simulink model "test_snap_dram_circ"  (Simulink 7.2)
settings: Solver=ode45  StartTime=0.0  StopTime=12000  RelTol=1e-3
libraries: xbsIndex_r4 x91, xps_library x7, casper_library_misc x5
settings Model: Creator=dsp  LastModifiedBy=root
settings OptimizationCC: InitFltsAndDblsToZero=on
settings DebuggingCC: SaveWithParameterizedLinksMsg=none  SignalResolutionControl=TryResolveAllWithWarning  MultiTaskDSMMsg=warning  MultiTaskCondExecSysMsg=none  StrictBusMsg=None
settings RTWCC: IncludeERTFirstTime=on
settings GRTTargetCC: TargetFcnLib=ansi_tfl_tmw.mat

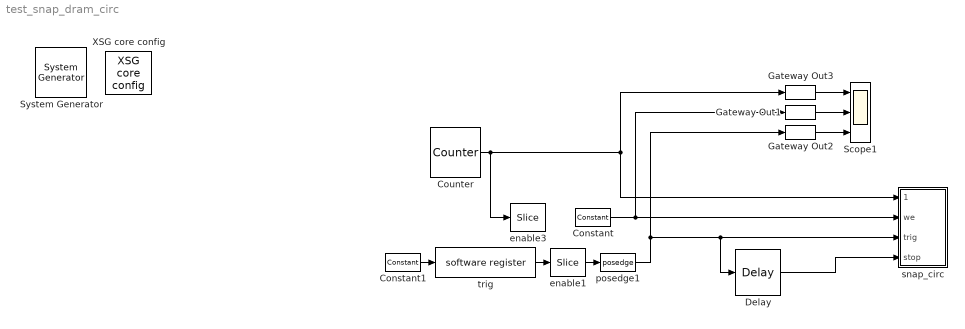
== system test_snap_dram_circ ==
  " System Generator" : xbsIndex_r4/ System Generator  Tag=genX  SystemSampleTime=-1  xilinxfamily=virtex5  part=xc5vsx95t  speed=-1  package=ff1136  synthesis_tool=XST  clock_wrapper=Clock Enables  directory=./test_snap_dram_circ/sysgen  testbench=off  simulink_period=1  sysclk_period=10  dcm_input_clock_period=100  incr_netlist=off  trim_vbits=Everywhere in SubSystem  dbl_ovrd=According to Block Masks  core_generation=According to Block Masks  run_coregen=off  deprecated_control=off  eval_field=0  block_type=sysgen
      settings: block_version=10.1.3
  Constant : xbsIndex_r4/Constant  arith_type=Boolean  const=1  n_bits=1  bin_pt=0  explicit_period=on  period=1  equ=P=C  opselect=C  inp2=PCIN>>17  opr=+  inp1=P  carry=CIN  dbl_ovrd=off  block_type=constant
  Constant1 : xbsIndex_r4/Constant  arith_type=Boolean  const=1  n_bits=1  bin_pt=0  explicit_period=on  period=1  equ=P=C  opselect=C  inp2=PCIN>>17  opr=+  inp1=P  carry=CIN  dbl_ovrd=off  block_type=constant
  Counter : xbsIndex_r4/Counter  cnt_type=Free Running  cnt_to=Inf  operation=Up  start_count=0  cnt_by_val=1  arith_type=Unsigned  n_bits=64  bin_pt=0  load_pin=off  rst=off  en=off  explicit_period=on  period=1  dbl_ovrd=off  use_behavioral_HDL=off  implementation=Fabric  use_rpm=on  block_type=counter
      settings: xl_area=[0, 0, 0, 0, 0, 0, 0]
  Delay : xbsIndex_r4/Delay  en=off  latency=5200  dbl_ovrd=off  reg_retiming=off  block_type=delay
      settings: xl_area=[0, 0, 0, 0, 0, 0, 0]
  Gateway Out1 : xbsIndex_r4/Gateway Out  hdl_port=off  timing_constraint=None  locs_specified=off  LOCs={}  block_type=gatewayout
      settings: infoedit="Gateway out block.  Converts Xilinx fixed point inputs into ouputs of type Simulink integer, double, or fixed point.<P><P>Hardware notes:  In hardware these blocks become top level output ports or are discarded, depending on how they are configured."  xl_area=[0, 0, 0, 0, 0, 0, 0]  block_version=10.1.3
  Gateway Out2 : xbsIndex_r4/Gateway Out  hdl_port=off  timing_constraint=None  locs_specified=off  LOCs={}  block_type=gatewayout
      settings: infoedit="Gateway out block.  Converts Xilinx fixed point inputs into ouputs of type Simulink integer, double, or fixed point.<P><P>Hardware notes:  In hardware these blocks become top level output ports or are discarded, depending on how they are configured."  xl_area=[0, 0, 0, 0, 0, 0, 0]  block_version=10.1.3
  Gateway Out3 : xbsIndex_r4/Gateway Out  hdl_port=off  timing_constraint=None  locs_specified=off  LOCs={}  block_type=gatewayout
      settings: infoedit="Gateway out block.  Converts Xilinx fixed point inputs into ouputs of type Simulink integer, double, or fixed point.<P><P>Hardware notes:  In hardware these blocks become top level output ports or are discarded, depending on how they are configured."  xl_area=[0, 0, 0, 0, 0, 0, 0]  block_version=10.1.3
  Scope1 : Scope  NumInputPorts=3
      settings: YMin=272014000~0~0  YMax=300648000~110~1
  XSG core config : xps_library/XSG core config  Tag=xps:xsg  SystemSampleTime=-1  hw_sys=ROACH:sx95t  ibob_linux=off  clk_src=sys_clk  iBOB_clk_src=sys_clk  BEE2_ctrl_clk_src=sys_clk  BEE2_usr_clk_src=sys_clk  ROACH_clk_src=sys_clk  CORR_clk_src=sys_clk  gpio_clk_io_group=iBOB:sma  gpio_clk_bit_index=0  clk_rate=100  sample_period=1  synthesis_tool=XST  mpc_type=powerpc440_ext
  enable1 : xbsIndex_r4/Slice  nbits=1  boolean_output=on  mode=Lower Bit Location + Width  bit1=0  base1=LSB of Input  bit0=0  base0=LSB of Input  dbl_ovrd=off  block_type=slice
      settings: infoedit="Extracts a given range of bits from each input sample and presents it at the output.  The output type is ordinarily unsigned with binary point at zero, but can be Boolean when the slice is one bit wide.<P><P>Hardware notes: In hardware this block costs nothing."  block_version=10.1.3
  enable3 : xbsIndex_r4/Slice  nbits=1  boolean_output=on  mode=Lower Bit Location + Width  bit1=0  base1=LSB of Input  bit0=0  base0=LSB of Input  dbl_ovrd=off  block_type=slice
      settings: infoedit="Extracts a given range of bits from each input sample and presents it at the output.  The output type is ordinarily unsigned with binary point at zero, but can be Boolean when the slice is one bit wide.<P><P>Hardware notes: In hardware this block costs nothing."  block_version=10.1.3
  posedge1 : casper_library_misc/posedge  Tag=Rising Edge Detector  SystemSampleTime=-1
  snap_circ : Subsystem  mask(snap_circ){nsamples=29}
      mask prompts: nsamples "Number of Samples (2^?)"
      mask help:
      | Backwards compatible with the normal snap block, but with the following upgrades:
      |  1) Ability to offset the trigger. Optionally delay the fabric trigger by a user-specified number of valids.
      |  2) 'Addr' register's MSb now indicates 'busy capturing'.
      |  3) Ability to capture continuously until a stop pulse is received. Data is captured into BRAM continuously, with old data being overwritten until a stop command is received. Then stop capturing when memory is filled. This enables you to get some data before and some data after the stop pulse. Use the 'tr_en_cnt' register to determine where you are in your vector.
  trig : xps_library/software register  Tag=xps:sw_reg  SystemSampleTime=-1  io_dir=From Processor  arith_type=Unsigned  bitwidth=32  bin_pt=0  sample_period=1  gw_name=test_snap_dram_circ_trig_user_data_out
      link override test_snap_circ_trig_user_data_out: arith_type=Unsigned  n_bits=32  bin_pt=0  period=1
  wires:
  Counter/1 -> Gateway Out3/1, snap_circ/1(data_in), enable3/1
  trig/1 -> enable1/1
  posedge1/1 -> Gateway Out2/1, Delay/1, snap_circ/3(trig)
  Gateway Out2/1 -> Scope1/3
  Gateway Out1/1 -> Scope1/2
  Gateway Out3/1 -> Scope1/1
  Constant1/1 -> trig/1
  enable1/1 -> posedge1/1
  Delay/1 -> snap_circ/4(stop)
  Constant/1 -> Gateway Out1/1, snap_circ/2(we)

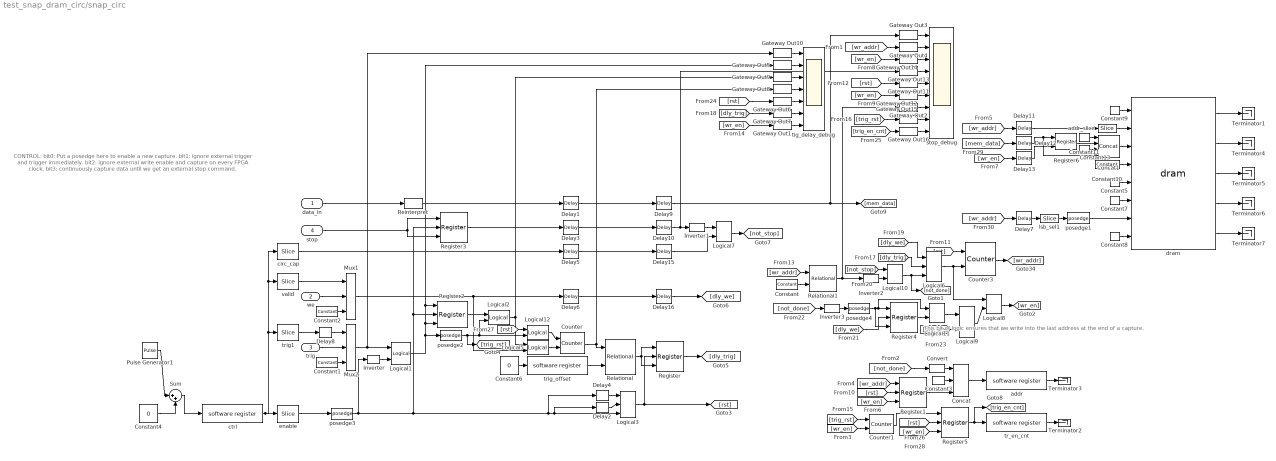
== system test_snap_dram_circ/snap_circ ==
  note: CONTROL:
      | bit0: Put a posedge here to enable a new capture.
      | bit1: ignore external trigger and trigger immediately.
      | bit2: ignore external write enable and capture on every FPGA clock.
      | bit3: continuously capture data until we get an external stop command.
  note: This bit of logic ensures that we
      | write into the last address
      | at the end of a capture.
  data_in : Inport  OutDataType=sfix(16)  OutScaling=2^0
  we : Inport  Port=2  OutDataType=sfix(16)  OutScaling=2^0
  trig : Inport  Port=3  OutDataType=sfix(16)  OutScaling=2^0
  stop : Inport  Port=4  OutDataType=sfix(16)  OutScaling=2^0
  Concat : xbsIndex_r4/Concat  num_inputs=3  dbl_ovrd=off  block_type=concat
      settings: block_version=10.1.3
  Concat1 : xbsIndex_r4/Concat  num_inputs=4  dbl_ovrd=off  block_type=concat
      settings: block_version=10.1.3
  Constant : xbsIndex_r4/Constant  arith_type=Unsigned  const=(2^nsamples)-1  n_bits=nsamples  bin_pt=0  explicit_period=on  period=1  equ=P=C  opselect=C  inp2=PCIN>>17  opr=+  inp1=P  carry=CIN  dbl_ovrd=off  block_type=constant
  Constant1 : xbsIndex_r4/Constant  arith_type=Boolean  const=1  n_bits=1  bin_pt=0  explicit_period=on  period=1  equ=P=C  opselect=C  inp2=PCIN>>17  opr=+  inp1=P  carry=CIN  dbl_ovrd=off  block_type=constant
  Constant10 : xbsIndex_r4/Constant  arith_type=Unsigned  const=2^32-1  n_bits=18  bin_pt=0  explicit_period=on  period=1  equ=P=C  opselect=C  inp2=PCIN>>17  opr=+  inp1=P  carry=CIN  dbl_ovrd=off  block_type=constant
  Constant11 : xbsIndex_r4/Constant  arith_type=Unsigned  const=0  n_bits=(144-128)/2  bin_pt=0  explicit_period=on  period=1  equ=P=C  opselect=C  inp2=PCIN>>17  opr=+  inp1=P  carry=CIN  dbl_ovrd=off  block_type=constant
  Constant13 : xbsIndex_r4/Constant  arith_type=Unsigned  const=0  n_bits=(144-128)/2  bin_pt=0  explicit_period=on  period=1  equ=P=C  opselect=C  inp2=PCIN>>17  opr=+  inp1=P  carry=CIN  dbl_ovrd=off  block_type=constant
  Constant2 : xbsIndex_r4/Constant  arith_type=Boolean  const=1  n_bits=1  bin_pt=0  explicit_period=on  period=1  equ=P=C  opselect=C  inp2=PCIN>>17  opr=+  inp1=P  carry=CIN  dbl_ovrd=off  block_type=constant
  Constant3 : xbsIndex_r4/Constant  arith_type=Unsigned  const=0  n_bits=32-nsamples-1  bin_pt=0  explicit_period=on  period=1  equ=P=C  opselect=C  inp2=PCIN>>17  opr=+  inp1=P  carry=CIN  dbl_ovrd=off  block_type=constant
  Constant4 : Constant  Value=0  OutDataType=sfix(16)  OutScaling=2^0
  Constant5 : xbsIndex_r4/Constant  arith_type=Boolean  const=0  n_bits=nsamples  bin_pt=0  explicit_period=on  period=1  equ=P=C  opselect=C  inp2=PCIN>>17  opr=+  inp1=P  carry=CIN  dbl_ovrd=off  block_type=constant
  Constant6 : Constant  Value=0  OutDataType=sfix(16)  OutScaling=2^0
  Constant7 : xbsIndex_r4/Constant  arith_type=Unsigned  const=0  n_bits=8  bin_pt=0  explicit_period=on  period=1  equ=P=C  opselect=C  inp2=PCIN>>17  opr=+  inp1=P  carry=CIN  dbl_ovrd=off  block_type=constant
  Constant8 : xbsIndex_r4/Constant  arith_type=Boolean  const=1  n_bits=nsamples  bin_pt=0  explicit_period=on  period=1  equ=P=C  opselect=C  inp2=PCIN>>17  opr=+  inp1=P  carry=CIN  dbl_ovrd=off  block_type=constant
  Constant9 : xbsIndex_r4/Constant  arith_type=Boolean  const=0  n_bits=nsamples  bin_pt=0  explicit_period=on  period=1  equ=P=C  opselect=C  inp2=PCIN>>17  opr=+  inp1=P  carry=CIN  dbl_ovrd=off  block_type=constant
  Convert : xbsIndex_r4/Convert  arith_type=Unsigned  n_bits=1  bin_pt=0  quantization=Truncate  overflow=Wrap  latency=0  dbl_ovrd=off  pipeline=off  block_type=convert
      settings: block_version=10.1.3
  Counter : xbsIndex_r4/Counter  cnt_type=Free Running  cnt_to=Inf  operation=Up  start_count=0  cnt_by_val=1  arith_type=Unsigned  n_bits=32  bin_pt=0  load_pin=off  rst=on  en=on  explicit_period=on  period=1  dbl_ovrd=off  use_behavioral_HDL=off  implementation=Fabric  use_rpm=on  block_type=counter
      settings: xl_area=[0, 0, 0, 0, 0, 0, 0]
  Counter1 : xbsIndex_r4/Counter  cnt_type=Free Running  cnt_to=Inf  operation=Up  start_count=0  cnt_by_val=1  arith_type=Unsigned  n_bits=32  bin_pt=0  load_pin=off  rst=on  en=on  explicit_period=on  period=1  dbl_ovrd=off  use_behavioral_HDL=off  implementation=Fabric  use_rpm=on  block_type=counter
      settings: xl_area=[0, 0, 0, 0, 0, 0, 0]
  Counter3 : xbsIndex_r4/Counter  cnt_type=Free Running  cnt_to=1  operation=Up  start_count=0  cnt_by_val=1  arith_type=Unsigned  n_bits=nsamples  bin_pt=0  load_pin=off  rst=on  en=on  explicit_period=on  period=1  dbl_ovrd=off  use_behavioral_HDL=off  implementation=Fabric  use_rpm=on  block_type=counter
      settings: xl_area=[0, 0, 0, 0, 0, 0, 0]
  Delay{1,3..7,9..13,15..16} (13 alike) : xbsIndex_r4/Delay  en=off  latency=1  dbl_ovrd=off  reg_retiming=on  block_type=delay
      settings: xl_area=[0, 0, 0, 0, 0, 0, 0]
  Delay2 : xbsIndex_r4/Delay  en=off  latency=2  dbl_ovrd=off  reg_retiming=on  block_type=delay
      settings: xl_area=[0, 0, 0, 0, 0, 0, 0]
  Delay8 : xbsIndex_r4/Delay  en=off  latency=3  dbl_ovrd=off  reg_retiming=on  block_type=delay
      settings: xl_area=[0, 0, 0, 0, 0, 0, 0]
  Gateway Out{1..16} (16 alike) : xbsIndex_r4/Gateway Out  hdl_port=off  timing_constraint=None  locs_specified=off  LOCs={}  block_type=gatewayout
      settings: infoedit="Gateway out block.  Converts Xilinx fixed point inputs into ouputs of type Simulink integer, double, or fixed point.<P><P>Hardware notes:  In hardware these blocks become top level output ports or are discarded, depending on how they are configured."  xl_area=[0, 0, 0, 0, 0, 0, 0]  block_version=10.1.3
  Inverter{,1..3} (4 alike) : xbsIndex_r4/Inverter  en=off  latency=0  dbl_ovrd=off  block_type=inv
      settings: xl_area=[0, 0, 0, 0, 0, 0, 0]
  Logical{1,5,7,9} (4 alike) : xbsIndex_r4/Logical  logical_function=AND  inputs=2  en=off  latency=0  precision=Full  arith_type=Unsigned  n_bits=8  bin_pt=2  align_bp=on  dbl_ovrd=off  block_type=logical
      settings: xl_area=[0, 0, 0, 0, 0, 0, 0]
  Logical{2,8,10..12} (5 alike) : xbsIndex_r4/Logical  logical_function=OR  inputs=2  en=off  latency=0  precision=Full  arith_type=Unsigned  n_bits=8  bin_pt=2  align_bp=on  dbl_ovrd=off  block_type=logical
      settings: xl_area=[0, 0, 0, 0, 0, 0, 0]
  Logical3 : xbsIndex_r4/Logical  logical_function=OR  inputs=3  en=off  latency=0  precision=Full  arith_type=Unsigned  n_bits=8  bin_pt=2  align_bp=on  dbl_ovrd=off  block_type=logical
      settings: xl_area=[0, 0, 0, 0, 0, 0, 0]
  Logical6 : xbsIndex_r4/Logical  logical_function=AND  inputs=3  en=off  latency=0  precision=Full  arith_type=Unsigned  n_bits=8  bin_pt=2  align_bp=on  dbl_ovrd=off  block_type=logical
      settings: xl_area=[0, 0, 0, 0, 0, 0, 0]
  Mux1 : xbsIndex_r4/Mux  inputs=2  en=off  latency=0  precision=Full  arith_type="Signed  (2's comp)"  n_bits=8  bin_pt=2  quantization=Truncate  overflow=Wrap  dbl_ovrd=off  block_type=mux
      settings: xl_area=[0, 0, 0, 0, 0, 0, 0]
  Mux2 : xbsIndex_r4/Mux  inputs=2  en=off  latency=0  precision=Full  arith_type="Signed  (2's comp)"  n_bits=8  bin_pt=2  quantization=Truncate  overflow=Wrap  dbl_ovrd=off  block_type=mux
      settings: xl_area=[0, 0, 0, 0, 0, 0, 0]
  Pulse Generator1 : DiscretePulseGenerator  Period=4096  PulseWidth=2
  Register{,1..5} (6 alike) : xbsIndex_r4/Register  init=0  rst=on  en=on  dbl_ovrd=off  block_type=register
      settings: xl_area=[0, 0, 0, 0, 0, 0, 0]
  Register6 : xbsIndex_r4/Register  init=0  rst=off  en=on  dbl_ovrd=off  block_type=register
  Reinterpret : xbsIndex_r4/Reinterpret  force_arith_type=on  arith_type=Unsigned  force_bin_pt=on  bin_pt=0  block_type=reinterpret
      settings: infoedit="Changes signal type without altering the binary representation.   You can changed the signal between signed and unsigned, and relocate the binary point.<P><P>Hardware notes: In hardware this block costs nothing.<P><P>Example:  Suppose the input is 6 bits wide, signed, with 2 fractional bits, and the output is forced to unsigned with 0 fractional bits.  Then an input of -2.0 (1110.00 in binary 2's complement) becomes an output of 56 (111000 in binary)."  block_version=10.1.3
  Relational : xbsIndex_r4/Relational  mode=a>b  en=off  latency=0  dbl_ovrd=off  block_type=relational
      settings: xl_area=[0, 0, 0, 0, 0, 0, 0]  block_version=10.1.3
  Relational1 : xbsIndex_r4/Relational  mode=a>=b  en=off  latency=0  dbl_ovrd=off  block_type=relational
      settings: xl_area=[0, 0, 0, 0, 0, 0, 0]  block_version=10.1.3
  Sum : Sum  Inputs=|++  OutDataType=sfix(16)  OutScaling=2^0
  Terminator{1..7} (7 alike) : Terminator
  addr : xps_library/software register  Tag=xps:sw_reg  SystemSampleTime=-1  io_dir=To Processor  arith_type=Unsigned  bitwidth=32  bin_pt=0  sample_period=1  gw_name=test_snap_dram_circ_snap_circ_addr_user_data_in
      link override convert: arith_type=Unsigned  n_bits=32  bin_pt=0
  addr_slice : xbsIndex_r4/Slice  nbits=72  boolean_output=off  mode=Two Bit Locations  bit1=0  base1=MSB of Input  bit0=2  base0=LSB of Input  dbl_ovrd=off  block_type=slice
      settings: block_version=10.1.3
  circ_cap : xbsIndex_r4/Slice  nbits=1  boolean_output=on  mode=Lower Bit Location + Width  bit1=0  base1=LSB of Input  bit0=3  base0=LSB of Input  dbl_ovrd=off  block_type=slice
      settings: infoedit="Extracts a given range of bits from each input sample and presents it at the output.  The output type is ordinarily unsigned with binary point at zero, but can be Boolean when the slice is one bit wide.<P><P>Hardware notes: In hardware this block costs nothing."  block_version=10.1.3
  ctrl : xps_library/software register  Tag=xps:sw_reg  SystemSampleTime=-1  io_dir=From Processor  arith_type=Unsigned  bitwidth=32  bin_pt=0  sample_period=1  gw_name=test_snap_dram_circ_snap_circ_ctrl_user_data_out
      link override r_4f_2x_16a_r322d_snap_descramble0_ctrl_user_data_out: arith_type=Unsigned  n_bits=32  bin_pt=0  period=1
      link override test_snap2_10_1_snap_circ_ctrl_user_data_out: arith_type=Unsigned  n_bits=32  bin_pt=0  period=1
      link override test_snap_circ_snap_circ_ctrl_user_data_out: arith_type=Unsigned  n_bits=32  bin_pt=0  period=1
  dram : xps_library/dram  Tag=xps:dram  SystemSampleTime=-1  dimm=1  arith_type=Unsigned  bin_pt=0  ip_clock=200  sample_period=1  bram_fifos=on  disable_tag=on  use_sim=off  ram_depth=18  bank_mgt=off  wide_data=off  half_burst=off  use_sniffer=on
      link override convert_data_in: arith_type=Unsigned  n_bits=144  bin_pt=0
      link override convert_wr_be: n_bits=18
      link override force_rd_dout: arith_type=Unsigned  bin_pt=0
      link override sim_wrapper/dram_sim: sim_method=Inactive  engine_block=ModelSim
      link override test_snap_dram_snap_circ_dram_Mem_Rd_Dout: n_bits=144
  enable : xbsIndex_r4/Slice  nbits=1  boolean_output=on  mode=Lower Bit Location + Width  bit1=0  base1=LSB of Input  bit0=0  base0=LSB of Input  dbl_ovrd=off  block_type=slice
      settings: infoedit="Extracts a given range of bits from each input sample and presents it at the output.  The output type is ordinarily unsigned with binary point at zero, but can be Boolean when the slice is one bit wide.<P><P>Hardware notes: In hardware this block costs nothing."  block_version=10.1.3
  lsb_sel1 : xbsIndex_r4/Slice  nbits=1  boolean_output=on  mode=Lower Bit Location + Width  bit1=0  base1=LSB of Input  bit0=0  base0=LSB of Input  dbl_ovrd=off  block_type=slice
      settings: infoedit="Extracts a given range of bits from each input sample and presents it at the output.  The output type is ordinarily unsigned with binary point at zero, but can be Boolean when the slice is one bit wide.<P><P>Hardware notes: In hardware this block costs nothing."  block_version=10.1.3
  posedge{1..4} (4 alike) : casper_library_misc/posedge  Tag=Rising Edge Detector  SystemSampleTime=-1
  stop_debug : Scope  NumInputPorts=9
      settings: YMin=2.72014e+008~0~0~-5~-5~-5~-5~-5~-5  YMax=3.00648e+008~110~1~5~5~5~5~5~5  SaveName=ScopeData12
  tig_delay_debug : Scope  NumInputPorts=7
      settings: YMin=2.72014e+008~0~0~-5~-5~-5~-5  YMax=3.00648e+008~110~1~5~5~5~5  SaveName=ScopeData16
  tr_en_cnt : xps_library/software register  Tag=xps:sw_reg  SystemSampleTime=-1  io_dir=To Processor  arith_type=Unsigned  bitwidth=32  bin_pt=0  sample_period=1  gw_name=test_snap_dram_circ_snap_circ_tr_en_cnt_user_data_in
      link override convert: arith_type=Unsigned  n_bits=32  bin_pt=0
  trig1 : xbsIndex_r4/Slice  nbits=1  boolean_output=on  mode=Lower Bit Location + Width  bit1=0  base1=LSB of Input  bit0=1  base0=LSB of Input  dbl_ovrd=off  block_type=slice
      settings: infoedit="Extracts a given range of bits from each input sample and presents it at the output.  The output type is ordinarily unsigned with binary point at zero, but can be Boolean when the slice is one bit wide.<P><P>Hardware notes: In hardware this block costs nothing."  block_version=10.1.3
  trig_offset : xps_library/software register  Tag=xps:sw_reg  SystemSampleTime=-1  io_dir=From Processor  arith_type=Unsigned  bitwidth=32  bin_pt=0  sample_period=1  gw_name=test_snap_dram_circ_snap_circ_trig_offset_user_data_out
      link override test_snap_circ_snap_circ_trig_offset_user_data_out: arith_type=Unsigned  n_bits=32  bin_pt=0  period=1
  valid : xbsIndex_r4/Slice  nbits=1  boolean_output=on  mode=Lower Bit Location + Width  bit1=0  base1=LSB of Input  bit0=2  base0=LSB of Input  dbl_ovrd=off  block_type=slice
      settings: infoedit="Extracts a given range of bits from each input sample and presents it at the output.  The output type is ordinarily unsigned with binary point at zero, but can be Boolean when the slice is one bit wide.<P><P>Hardware notes: In hardware this block costs nothing."  block_version=10.1.3
  wires:
  data_in/1 -> Reinterpret/1
  valid/1 -> Mux1/1
  trig1/1 -> Delay8/1
  Constant2/1 -> Mux1/3
  we/1 -> Mux1/2
  Constant1/1 -> Mux2/3
  ctrl/1 -> trig1/1, valid/1, circ_cap/1, enable/1
  enable/1 -> posedge3/1
  trig/1 -> Mux2/2
  Constant4/1 -> Sum/2
  Sum/1 -> ctrl/1
  Pulse Generator1/1 -> Sum/1
  Mux2/1 -> Logical1/1, Gateway Out10/1
  Inverter/1 -> Logical1/2
  Mux1/1 -> Logical5/2, Delay6/1
  posedge3/1 -> Inverter/1, Delay4/1, Delay2/1, Logical3/3, Register2/2, Register3/2
  Logical1/1 -> Register2/1, Gateway Out5/1, Register2/3, posedge2/1
  Register2/1 -> Logical2/1
  Delay4/1 -> Logical3/1
  Constant6/1 -> trig_offset/1
  trig_offset/1 -> Relational/2
  Relational/1 -> Register/3, Register/1
  Logical2/1 -> Logical5/1, Gateway Out9/1
  Counter/1 -> Gateway Out8/1, Relational/1
  Delay2/1 -> Logical3/2
  Gateway Out9/1 -> tig_delay_debug/3
  Gateway Out5/1 -> tig_delay_debug/2
  Gateway Out8/1 -> tig_delay_debug/4
  Gateway Out6/1 -> tig_delay_debug/5
  Gateway Out10/1 -> tig_delay_debug/1
  Gateway Out7/1 -> tig_delay_debug/6
  Gateway Out1/1 -> tig_delay_debug/7
  Reinterpret/1 -> Delay1/1
  Logical6/1 -> Counter3/2, Logical8/1
  Counter3/1 -> [wr_addr]
  Constant/1 -> Relational1/2
  Register3/1 -> Delay3/1
  Inverter1/1 -> Logical7/1
  Gateway Out14/1 -> stop_debug/3
  Gateway Out4/1 -> stop_debug/2
  Gateway Out13/1 -> stop_debug/4
  Gateway Out11/1 -> stop_debug/5
  Gateway Out3/1 -> stop_debug/1
  Gateway Out12/1 -> stop_debug/6
  Gateway Out2/1 -> stop_debug/7
  Logical3/1 -> Register/2, [rst]
  Logical10/1 -> Logical6/3, [not_done]
  Inverter2/1 -> Logical10/2
  Delay11/1 -> addr_slice/1
  Delay13/1 -> Register6/2
  Concat/1 -> addr/1
  stop/1 -> Register3/1, Register3/3
  circ_cap/1 -> Delay5/1
  Convert/1 -> Concat/1
  Constant3/1 -> Concat/2
  tr_en_cnt/1 -> Terminator2/1
  addr/1 -> Terminator3/1
  Delay9/1 -> Gateway Out3/1, [mem_data]
  Delay10/1 -> Inverter1/1, Gateway Out13/1
  Delay15/1 -> Logical7/2
  Logical5/1 -> Counter/2
  Register1/1 -> Concat/3
  [wr_addr] -> Delay11/1
  [wr_addr] -> Gateway Out4/1
  [not_done] -> Convert/1
  [wr_en] -> Counter1/2
  [wr_addr] -> Register1/1
  [wr_en] -> Register1/3
  [wr_en] -> Delay13/1
  [wr_en] -> Gateway Out14/1
  [wr_en] -> Gateway Out12/1
  [rst] -> Register1/2
  [rst] -> Counter3/1
  [rst] -> Gateway Out11/1
  Relational1/1 -> Gateway Out2/1, Inverter2/1
  [wr_addr] -> Relational1/1
  [wr_en] -> Gateway Out1/1
  [trig_rst] -> Counter1/1
  Gateway Out15/1 -> stop_debug/8
  [trig_rst] -> Gateway Out15/1
  Register/1 -> [dly_trig]
  [dly_trig] -> Gateway Out7/1
  Delay16/1 -> [dly_we]
  [dly_we] -> Logical6/1
  [dly_trig] -> Logical6/2
  Logical7/1 -> [not_stop]
  [not_stop] -> Logical10/1
  Logical8/1 -> [wr_en]
  [not_done] -> Inverter3/1
  Inverter3/1 -> posedge4/1
  posedge4/1 -> Register4/3, Register4/1, Logical11/1
  [dly_we] -> Register4/2
  [dly_we] -> Logical9/2
  Logical9/1 -> Logical8/2
  Logical11/1 -> Logical9/1
  Register4/1 -> Logical11/2
  [rst] -> Gateway Out6/1
  Delay8/1 -> Mux2/1
  [trig_en_cnt] -> Gateway Out16/1
  Gateway Out16/1 -> stop_debug/9
  Counter1/1 -> Register5/1
  [wr_en] -> Register5/3
  [rst] -> Register5/2
  Register5/1 -> tr_en_cnt/1, [trig_en_cnt]
  Logical12/1 -> Counter/1
  [rst] -> Logical12/1
  posedge2/1 -> Logical2/2, Logical12/2, [trig_rst]
  Delay1/1 -> Delay9/1
  Delay3/1 -> Delay10/1
  Delay5/1 -> Delay15/1
  Delay6/1 -> Delay16/1
  Constant5/1 -> dram/5
  Constant7/1 -> dram/6
  Constant8/1 -> dram/8
  Constant9/1 -> dram/1
  addr_slice/1 -> dram/2
  Register6/1 -> Concat1/2
  Concat1/1 -> dram/3
  Constant10/1 -> dram/4
  posedge1/1 -> dram/7
  dram/1 -> Terminator1/1
  dram/2 -> Terminator4/1
  dram/3 -> Terminator5/1
  dram/4 -> Terminator6/1
  dram/5 -> Terminator7/1
  lsb_sel1/1 -> posedge1/1
  Delay12/1 -> Register6/1, Concat1/4
  [mem_data] -> Delay12/1
  [wr_addr] -> Delay7/1
  Delay7/1 -> lsb_sel1/1
  Constant11/1 -> Concat1/1
  Constant13/1 -> Concat1/3
